simulink model "NarwhaleSimscape"  (R2021b)
settings: Solver=VariableStepAuto  StartTime=0.0  StopTime=12  FixedStep=10^-3  RelTol=1e-3
undefined symbols (not defined in the file): X, Y, Z
libraries: nesl_utility x34, sm_lib x28, slpidlib x5
(part 1 of 3)
settings Model: Creator=matas  LastModifiedBy=matas
settings SolverCC: AlgebraicLoopSolver=TrustRegion
settings DebuggingCC: SFMachineParentedDataDiag=warning

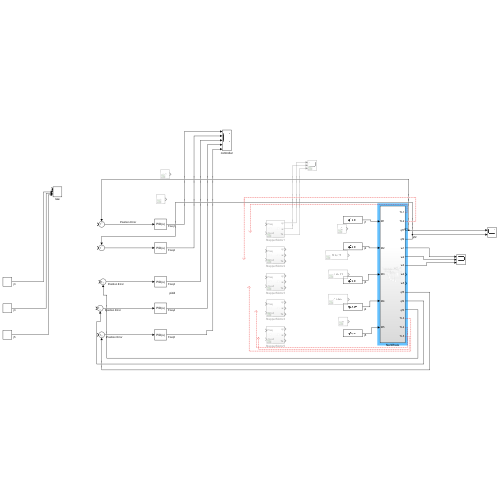
[thumbnail: Simulink's stored preview of the top-level diagram]
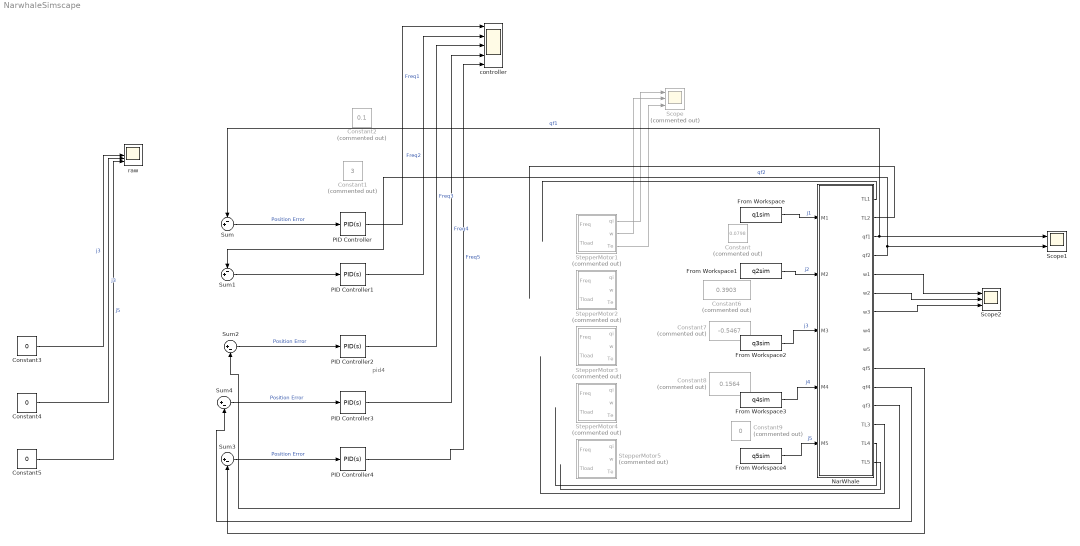
== system NarwhaleSimscape ==
  note: pid4
  Constant : Constant  Commented=on  Value=0.0798
  Constant1 : Constant  Commented=on  Value=3
  Constant2 : Constant  Commented=on  Value=0.1
  Constant3 : Constant  Value=0
  Constant4 : Constant  Value=0
  Constant5 : Constant  Value=0
  Constant6 : Constant  Commented=on  Value=0.3903
  Constant7 : Constant  Commented=on  Value=-0.5467
  Constant8 : Constant  Commented=on  Value=0.1564
  Constant9 : Constant  Commented=on  Value=0
  From Workspace : FromWorkspace  VariableName=q1sim
  From Workspace1 : FromWorkspace  VariableName=q2sim
  From Workspace2 : FromWorkspace  VariableName=q3sim
  From Workspace3 : FromWorkspace  VariableName=q4sim
  From Workspace4 : FromWorkspace  VariableName=q5sim
  NarWhale : Subsystem
  PID Controller : slpidlib/PID Controller  Controller=PID  Form=Parallel  TimeDomain=Continuous-time  UseExternalTs=off  SampleTime=-1  IntegratorMethod=Forward Euler  FilterMethod=Forward Euler  ControllerParametersSource=internal  P=8  I=1  D=0.05  UseFilter=on  N=100  TunerSelectOption=Transfer Function Based (PID Tuner App)  InitialConditionSource=internal  InitialConditionForIntegrator=0  InitialConditionForFilter=0  DifferentiatorICPrevScaledInput=0  ExternalReset=none  TrackingMode=off  Kt=1  LimitOutput=off  SatLimitsSource=internal  UpperSaturationLimit=inf  LowerSaturationLimit=-inf  LinearizeAsGain=on  AntiWindupMode=none  Kb=1  POutMin=[]  POutMax=[]  IOutMin=[]  IOutMax=[]  DOutMin=[]  DOutMax=[]  NOutMin=[]  NOutMax=[]  SumOutMin=[]  SumOutMax=[]  SaturationOutMin=[]  SaturationOutMax=[]  PParamMin=[]  PParamMax=[]  IParamMin=[]  IParamMax=[]  DParamMin=[]  DParamMax=[]  NParamMin=[]  NParamMax=[]  KbParamMin=[]  KbParamMax=[]  KtParamMin=[]  KtParamMax=[]  KbOutMin=[]  KbOutMax=[]  KtOutMin=[]  KtOutMax=[]  IntegratorOutMin=[]  IntegratorOutMax=[]  FilterOutMin=[]  FilterOutMax=[]  SumI1OutMin=[]  SumI1OutMax=[]  SumI2OutMin=[]  SumI2OutMax=[]  SumI3OutMin=[]  SumI3OutMax=[]  SumI4OutMin=[]  SumI4OutMax=[]  SumDOutMin=[]  SumDOutMax=[]  DifferentiatorOutMin=[]  DifferentiatorOutMax=[]  FilterDiffOutCoefMin=[]  FilterDiffOutCoefMax=[]  ReciprocalOutMin=[]  ReciprocalOutMax=[]  SumDenOutMin=[]  SumDenOutMax=[]  SumNumOutMin=[]  SumNumOutMax=[]  DivideOutMin=[]  DivideOutMax=[]  UdiffTsProdOutMin=[]  UdiffTsProdOutMax=[]  NTsProdOutMin=[]  NTsProdOutMax=[]  UintegralTsProdOutMin=[]  UintegralTsProdOutMax=[]  UngainTsProdOutMin=[]  UngainTsProdOutMax=[]  IntegratorContinuousStateAttributes=''  IntegratorStateMustResolveToSignalObject=off  IntegratorRTWStateStorageClass=Auto  FilterContinuousStateAttributes=''  FilterStateMustResolveToSignalObject=off  FilterRTWStateStorageClass=Auto  ParallelPVariant=InternalParameters  IdealPVariant=Disabled  IVariant=InternalParameters  DVariant=InternalParameters  IntegratorVariant=Continuous  SatVariant=Disabled  AWVariant=Passthrough  PCopyVariant=Disabled  TRVariant=Disabled  FdbkBlocksVariant=Forward  IdealPFdbkVariant=Disabled  SatFdbkVariant=Disabled  DerivativeFilterVariant=ContFilter  NVariant=InternalParameters  NCopyVariant=Disabled  FilterICVariant=InternalICsFilter  IntegratorICVariant=InternalICs  ExternalResetVariant=Disabled  TRSumVariant=Passthrough  SumFdbkVariant=Disabled  SumVariant=Sum_PID  TsampFilterVariant=InternalTs  TsampNgainVariant=Passthrough  TsampIntegralVariant=Passthrough  ExternalSaturationOutDataTypeStr=Inherit: Same as second input
  PID Controller{1..4} (4 alike) : slpidlib/PID Controller  Controller=PID  Form=Parallel  TimeDomain=Continuous-time  UseExternalTs=off  SampleTime=-1  IntegratorMethod=Forward Euler  FilterMethod=Forward Euler  ControllerParametersSource=internal  P=8  I=1  D=0.5  UseFilter=on  N=100  TunerSelectOption=Transfer Function Based (PID Tuner App)  InitialConditionSource=internal  InitialConditionForIntegrator=0  InitialConditionForFilter=0  DifferentiatorICPrevScaledInput=0  ExternalReset=none  TrackingMode=off  Kt=1  LimitOutput=off  SatLimitsSource=internal  UpperSaturationLimit=inf  LowerSaturationLimit=-inf  LinearizeAsGain=on  AntiWindupMode=none  Kb=1  POutMin=[]  POutMax=[]  IOutMin=[]  IOutMax=[]  DOutMin=[]  DOutMax=[]  NOutMin=[]  NOutMax=[]  SumOutMin=[]  SumOutMax=[]  SaturationOutMin=[]  SaturationOutMax=[]  PParamMin=[]  PParamMax=[]  IParamMin=[]  IParamMax=[]  DParamMin=[]  DParamMax=[]  NParamMin=[]  NParamMax=[]  KbParamMin=[]  KbParamMax=[]  KtParamMin=[]  KtParamMax=[]  KbOutMin=[]  KbOutMax=[]  KtOutMin=[]  KtOutMax=[]  IntegratorOutMin=[]  IntegratorOutMax=[]  FilterOutMin=[]  FilterOutMax=[]  SumI1OutMin=[]  SumI1OutMax=[]  SumI2OutMin=[]  SumI2OutMax=[]  SumI3OutMin=[]  SumI3OutMax=[]  SumI4OutMin=[]  SumI4OutMax=[]  SumDOutMin=[]  SumDOutMax=[]  DifferentiatorOutMin=[]  DifferentiatorOutMax=[]  FilterDiffOutCoefMin=[]  FilterDiffOutCoefMax=[]  ReciprocalOutMin=[]  ReciprocalOutMax=[]  SumDenOutMin=[]  SumDenOutMax=[]  SumNumOutMin=[]  SumNumOutMax=[]  DivideOutMin=[]  DivideOutMax=[]  UdiffTsProdOutMin=[]  UdiffTsProdOutMax=[]  NTsProdOutMin=[]  NTsProdOutMax=[]  UintegralTsProdOutMin=[]  UintegralTsProdOutMax=[]  UngainTsProdOutMin=[]  UngainTsProdOutMax=[]  IntegratorContinuousStateAttributes=''  IntegratorStateMustResolveToSignalObject=off  IntegratorRTWStateStorageClass=Auto  FilterContinuousStateAttributes=''  FilterStateMustResolveToSignalObject=off  FilterRTWStateStorageClass=Auto  ParallelPVariant=InternalParameters  IdealPVariant=Disabled  IVariant=InternalParameters  DVariant=InternalParameters  IntegratorVariant=Continuous  SatVariant=Disabled  AWVariant=Passthrough  PCopyVariant=Disabled  TRVariant=Disabled  FdbkBlocksVariant=Forward  IdealPFdbkVariant=Disabled  SatFdbkVariant=Disabled  DerivativeFilterVariant=ContFilter  NVariant=InternalParameters  NCopyVariant=Disabled  FilterICVariant=InternalICsFilter  IntegratorICVariant=InternalICs  ExternalResetVariant=Disabled  TRSumVariant=Passthrough  SumFdbkVariant=Disabled  SumVariant=Sum_PID  TsampFilterVariant=InternalTs  TsampNgainVariant=Passthrough  TsampIntegralVariant=Passthrough  ExternalSaturationOutDataTypeStr=Inherit: Same as second input
  Scope : Scope  Commented=on  NumInputPorts=3
  Scope1 : Scope  NumInputPorts=2
  Scope2 : Scope  NumInputPorts=3
  StepperMotor1 : Subsystem  Commented=on
  StepperMotor2 : Subsystem  Commented=on
  StepperMotor3 : Subsystem  Commented=on
  StepperMotor4 : Subsystem  Commented=on
  StepperMotor5 : Subsystem  Commented=on
  Sum : Sum  Inputs=-+|
  Sum1 : Sum  Inputs=-+|
  Sum2 : Sum  Inputs=|+-
  Sum3 : Sum  Inputs=|+-
  Sum4 : Sum  Inputs=|+-
  controller : Scope  NumInputPorts=5
  raw : Scope  NumInputPorts=5
  wires:
  StepperMotor1/1(qi) -> Scope/1
  StepperMotor1/2(w) -> Scope/2
  StepperMotor1/3(Te) -> Scope/3
  NarWhale/1(TL1) -> ?
  NarWhale/3(qf1) -> Sum/1, Scope1/1  "qf1"
  Sum/1 -> PID Controller/1  "Position Error"
  PID Controller/1 -> controller/1  "Freq1"
  PID Controller1/1 -> controller/2  "Freq2"
  Sum1/1 -> PID Controller1/1
  NarWhale/4(qf2) -> Scope1/2, Sum1/1  "qf2"
  NarWhale/2(TL2) -> ?
  Sum2/1 -> PID Controller2/1  "Position Error"
  PID Controller2/1 -> controller/3  "Freq3"
  Constant3/1 -> raw/3  "j3"
  Sum4/1 -> PID Controller3/1  "Position Error"
  PID Controller3/1 -> controller/4  "Freq4"
  NarWhale/12(qf3) -> Sum2/2
  NarWhale/11(qf4) -> Sum4/2
  NarWhale/13(TL3) -> ?
  NarWhale/14(TL4) -> ?
  NarWhale/15(TL5) -> ?
  Constant5/1 -> raw/5  "j5"
  Sum3/1 -> PID Controller4/1  "Position Error"
  PID Controller4/1 -> controller/5  "Freq5"
  NarWhale/10(qf5) -> Sum3/2
  Constant4/1 -> raw/4  "j3"
  NarWhale/5(w1) -> Scope2/1
  NarWhale/6(w2) -> Scope2/2
  NarWhale/7(w3) -> Scope2/3
  From Workspace/1 -> NarWhale/1(M1)  "j1"
  From Workspace1/1 -> NarWhale/2(M2)  "j2"
  From Workspace2/1 -> NarWhale/3(M3)  "j3"
  From Workspace3/1 -> NarWhale/4(M4)  "j4"
  From Workspace4/1 -> NarWhale/5(M5)  "j5"

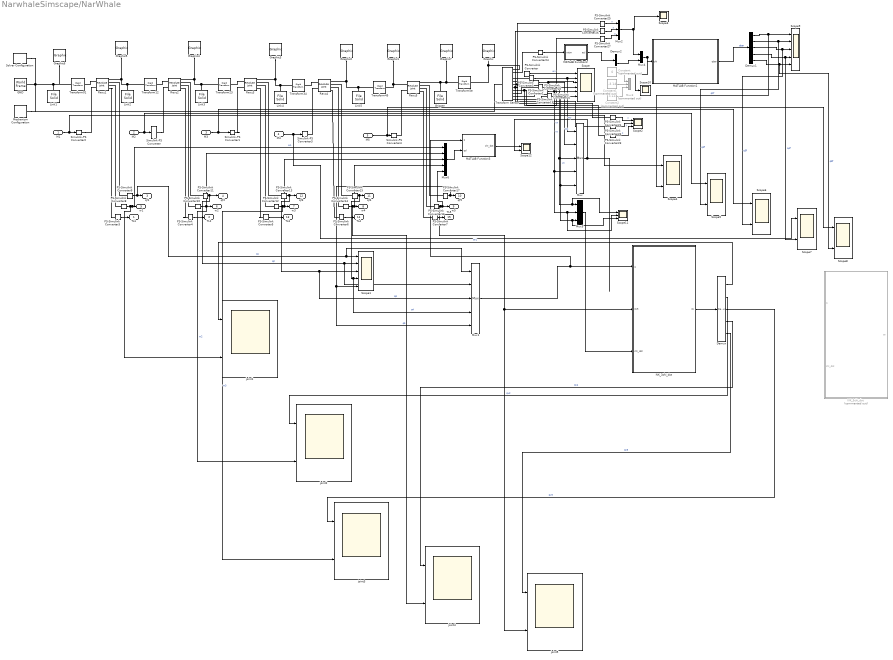
== system NarwhaleSimscape/NarWhale ==
  M1 : Inport
  M2 : Inport  Port=2
  M3 : Inport  Port=3
  M4 : Inport  Port=4
  M5 : Inport  Port=5
  Constant : Constant  Commented=on  Value=0
  Constant1 : Constant  Commented=on  Value=-3.14
  Constant2 : Constant  Commented=on  Value=3.14
  Demux : Demux  Outputs=5
  Demux1 : Demux  Outputs=5
  Demux2 : Demux  Outputs=3
  GND : sm_lib/Frames and Transforms/World Frame
  Graphic : sm_lib/Body Elements/Graphic  GraphicType=Marker  MarkerShape=Frame  MarkerSize=30  GraphicVisPropType=SimpleVisualProperties  GraphicDiffuseColor=[1.0 0.0 0.2]  GraphicSpecularColor=[0.5 0.5 0.5 1.0]  GraphicAmbientColor=[0.15 0.15 0.15 1.0]  GraphicEmissiveColor=[0.0 0.0 0.0 1.0]  GraphicShininess=75  GraphicOpacity=1.0
  Graphic1 : sm_lib/Body Elements/Graphic  GraphicType=Marker  MarkerShape=Frame  MarkerSize=30  GraphicVisPropType=SimpleVisualProperties  GraphicDiffuseColor=[1.0 1.0 0.2]  GraphicSpecularColor=[0.5 0.5 0.5 1.0]  GraphicAmbientColor=[0.15 0.15 0.15 1.0]  GraphicEmissiveColor=[0.0 0.0 0.0 1.0]  GraphicShininess=75  GraphicOpacity=1.0
  Graphic2 : sm_lib/Body Elements/Graphic  GraphicType=Marker  MarkerShape=Frame  MarkerSize=30  GraphicVisPropType=SimpleVisualProperties  GraphicDiffuseColor=[0.2 1.0 0.2]  GraphicSpecularColor=[0.5 0.5 0.5 1.0]  GraphicAmbientColor=[0.15 0.15 0.15 1.0]  GraphicEmissiveColor=[0.0 0.0 0.0 1.0]  GraphicShininess=75  GraphicOpacity=1.0
  Graphic3 : sm_lib/Body Elements/Graphic  GraphicType=Marker  MarkerShape=Frame  MarkerSize=30  GraphicVisPropType=SimpleVisualProperties  GraphicDiffuseColor=[0.2 0.2 1.0]  GraphicSpecularColor=[0.5 0.5 0.5 1.0]  GraphicAmbientColor=[0.15 0.15 0.15 1.0]  GraphicEmissiveColor=[0.0 0.0 0.0 1.0]  GraphicShininess=75  GraphicOpacity=1.0
  Graphic4 : sm_lib/Body Elements/Graphic  GraphicType=Marker  MarkerShape=Frame  MarkerSize=30  GraphicVisPropType=SimpleVisualProperties  GraphicDiffuseColor=[0.6 0.0 1.0]  GraphicSpecularColor=[0.5 0.5 0.5 1.0]  GraphicAmbientColor=[0.15 0.15 0.15 1.0]  GraphicEmissiveColor=[0.0 0.0 0.0 1.0]  GraphicShininess=75  GraphicOpacity=1.0
  Graphic5 : sm_lib/Body Elements/Graphic  GraphicType=Marker  MarkerShape=Frame  MarkerSize=30  GraphicVisPropType=SimpleVisualProperties  GraphicDiffuseColor=[1.0 1.0 1.0]  GraphicSpecularColor=[0.5 0.5 0.5 1.0]  GraphicAmbientColor=[0.15 0.15 0.15 1.0]  GraphicEmissiveColor=[0.0 0.0 0.0 1.0]  GraphicShininess=75  GraphicOpacity=1.0
  Graphic6 : sm_lib/Body Elements/Graphic  GraphicType=Marker  MarkerShape=Frame  MarkerSize=30  GraphicVisPropType=SimpleVisualProperties  GraphicDiffuseColor=[1.0 0.0 1.0]  GraphicSpecularColor=[0.5 0.5 0.5 1.0]  GraphicAmbientColor=[0.15 0.15 0.15 1.0]  GraphicEmissiveColor=[0.0 0.0 0.0 1.0]  GraphicShininess=75  GraphicOpacity=1.0
  Graphic7 : sm_lib/Body Elements/Graphic  GraphicType=Marker  MarkerShape=Frame  MarkerSize=30  GraphicVisPropType=SimpleVisualProperties  GraphicDiffuseColor=[0.4941 0.1843 0.5569]  GraphicSpecularColor=[0.5 0.5 0.5 1.0]  GraphicAmbientColor=[0.15 0.15 0.15 1.0]  GraphicEmissiveColor=[0.0 0.0 0.0 1.0]  GraphicShininess=75  GraphicOpacity=1.0
  Gripper : sm_lib/Body Elements/File Solid  ExtGeomFileName=C:\Users\matas\Documents\GitHub\Module89-Frab5-G3\Matlabscript_simscape\Simscape\NarwhaleCAD\GripperASM.STL  UnitType=Custom  ExtGeomFileUnits=mm  StepReaderType=HEX  ExportConvexHullGeometry=off  InertiaType=Custom  Mass=0.69041  MassUnits=kg  CenterOfMass=[3.8 0.1 197.24]  CenterOfMassUnits=mm  MomentsOfInertia=[17952.2303 19894.8925 4557.2173]  MomentsOfInertiaUnits=g*cm^2  ProductsOfInertia="[-45.0059 -1280.1589  8.8427]"  ProductsOfInertiaUnits=g*cm^2  BasedOnType=DensityFromFile  Density=1000  DensityUnits=kg/m^3  DoExposeReferenceFrame=on  SerializedFrames=<Frames/>  GraphicType=FromGeometry  MarkerShape=Sphere  MarkerSize=10  GraphicVisPropType=SimpleVisualProperties  GraphicDiffuseColor=[0.5 0.5 0.5]  GraphicSpecularColor=[0.5 0.5 0.5 1.0]  GraphicAmbientColor=[0.15 0.15 0.15 1.0]  GraphicEmissiveColor=[0.0 0.0 0.0 1.0]  GraphicShininess=75  GraphicOpacity=1.0
  IVK_3chi_dot : MATLAB Function  TreatAsAtomicUnit=on
  IVK_5chi_dot : MATLAB Function  Commented=on  TreatAsAtomicUnit=on
  Link1 : sm_lib/Body Elements/File Solid  ExtGeomFileName=C:\Users\matas\Documents\GitHub\Module89-Frab5-G3\Matlabscript_simscape\Simscape\NarwhaleCAD\asm_J1.STL  UnitType=Custom  ExtGeomFileUnits=mm  StepReaderType=HEX  ExportConvexHullGeometry=off  InertiaType=Custom  Mass=4.4  MassUnits=kg  CenterOfMass=[-62.94 0.00 77.26]  CenterOfMassUnits=mm  MomentsOfInertia=[233653.95 370833.8212 478183.0941]  MomentsOfInertiaUnits=g*cm^2  ProductsOfInertia=[-8.5995 11773.7055 -0.9031]  ProductsOfInertiaUnits=g*cm^2  BasedOnType=DensityFromFile  Density=1000  DensityUnits=kg/m^3  DoExposeReferenceFrame=on  SerializedFrames=<Frames/>  GraphicType=FromGeometry  MarkerShape=Sphere  MarkerSize=10  GraphicVisPropType=SimpleVisualProperties  GraphicDiffuseColor=[0.5 0.5 0.5]  GraphicSpecularColor=[0.5 0.5 0.5 1.0]  GraphicAmbientColor=[0.15 0.15 0.15 1.0]  GraphicEmissiveColor=[0.0 0.0 0.0 1.0]  GraphicShininess=75  GraphicOpacity=1.0
  Link2 : sm_lib/Body Elements/File Solid  ExtGeomFileName=C:\Users\matas\Documents\GitHub\Module89-Frab5-G3\Matlabscript_simscape\Simscape\NarwhaleCAD\link1.STL  UnitType=Custom  ExtGeomFileUnits=mm  StepReaderType=HEX  ExportConvexHullGeometry=off  InertiaType=Custom  Mass=3.0358  MassUnits=kg  CenterOfMass=[-43.29 -2.02 -88.16]  CenterOfMassUnits=mm  MomentsOfInertia=[97169.4169 112815.4665 119641.6148]  MomentsOfInertiaUnits=g*cm^2  ProductsOfInertia=[13604.2243 136476.2489 6464.8471]  ProductsOfInertiaUnits=g*cm^2  BasedOnType=DensityFromFile  Density=1000  DensityUnits=kg/m^3  DoExposeReferenceFrame=on  SerializedFrames=<Frames/>  GraphicType=FromGeometry  MarkerShape=Sphere  MarkerSize=10  GraphicVisPropType=FromFileVisualProperties  GraphicDiffuseColor=[0.5 0.5 0.5]  GraphicSpecularColor=[0.5 0.5 0.5 1.0]  GraphicAmbientColor=[0.15 0.15 0.15 1.0]  GraphicEmissiveColor=[0.0 0.0 0.0 1.0]  GraphicShininess=75  GraphicOpacity=1.0
  Link3 : sm_lib/Body Elements/File Solid  ExtGeomFileName=C:\Users\matas\Documents\GitHub\Module89-Frab5-G3\Matlabscript_simscape\Simscape\NarwhaleCAD\link2.STL  UnitType=Custom  ExtGeomFileUnits=mm  StepReaderType=HEX  ExportConvexHullGeometry=off  InertiaType=Custom  Mass=2.0778  MassUnits=kg  CenterOfMass=[162 -0.02 8.59]  CenterOfMassUnits=mm  MomentsOfInertia=[24739.1072 311541.7518 294173.41]  MomentsOfInertiaUnits=g*cm^2  ProductsOfInertia=[-387.45 21752.3776 353.8205]  ProductsOfInertiaUnits=g*cm^2  BasedOnType=DensityFromFile  Density=1000  DensityUnits=kg/m^3  DoExposeReferenceFrame=on  SerializedFrames=<Frames/>  GraphicType=FromGeometry  MarkerShape=Sphere  MarkerSize=10  GraphicVisPropType=FromFileVisualProperties  GraphicDiffuseColor=[0.5 0.5 0.5]  GraphicSpecularColor=[0.5 0.5 0.5 1.0]  GraphicAmbientColor=[0.15 0.15 0.15 1.0]  GraphicEmissiveColor=[0.0 0.0 0.0 1.0]  GraphicShininess=75  GraphicOpacity=1.0
  Link4 : sm_lib/Body Elements/File Solid  ExtGeomFileName=C:\Users\matas\Documents\GitHub\Module89-Frab5-G3\Matlabscript_simscape\Simscape\NarwhaleCAD\link3.STL  UnitType=Custom  ExtGeomFileUnits=mm  StepReaderType=HEX  ExportConvexHullGeometry=off  InertiaType=Custom  Mass=1.43881  MassUnits=kg  CenterOfMass=[-175.56 0.06 -6.33]  CenterOfMassUnits=mm  MomentsOfInertia=[16069.2959 173755.3840 164253.8860]  MomentsOfInertiaUnits=g*cm^2  ProductsOfInertia="[-41.6776 3243.5212  -172.4909]"  ProductsOfInertiaUnits=g*cm^2  BasedOnType=DensityFromFile  Density=1000  DensityUnits=kg/m^3  DoExposeReferenceFrame=on  SerializedFrames=<Frames/>  GraphicType=FromGeometry  MarkerShape=Sphere  MarkerSize=10  GraphicVisPropType=FromFileVisualProperties  GraphicDiffuseColor=[0.5 0.5 0.5]  GraphicSpecularColor=[0.5 0.5 0.5 1.0]  GraphicAmbientColor=[0.15 0.15 0.15 1.0]  GraphicEmissiveColor=[0.0 0.0 0.0 1.0]  GraphicShininess=75  GraphicOpacity=1.0
  Link5 : sm_lib/Body Elements/File Solid  ExtGeomFileName=C:\Users\matas\Documents\GitHub\Module89-Frab5-G3\Matlabscript_simscape\Simscape\NarwhaleCAD\J5_Asm.STL  UnitType=Custom  ExtGeomFileUnits=mm  StepReaderType=HEX  ExportConvexHullGeometry=off  InertiaType=Custom  Mass=0.354  MassUnits=kg  CenterOfMass=[-1.28 49.13 0.00]  CenterOfMassUnits=mm  MomentsOfInertia=[6817.7645 2848.9265 5884.7291]  MomentsOfInertiaUnits=g*cm^2  ProductsOfInertia="[-0.2087 1.8247  -13.0414]"  ProductsOfInertiaUnits=g*cm^2  BasedOnType=DensityFromFile  Density=1000  DensityUnits=kg/m^3  DoExposeReferenceFrame=on  SerializedFrames=<Frames/>  GraphicType=FromGeometry  MarkerShape=Sphere  MarkerSize=10  GraphicVisPropType=SimpleVisualProperties  GraphicDiffuseColor=[0.5 0.5 0.5]  GraphicSpecularColor=[0.5 0.5 0.5 1.0]  GraphicAmbientColor=[0.15 0.15 0.15 1.0]  GraphicEmissiveColor=[0.0 0.0 0.0 1.0]  GraphicShininess=75  GraphicOpacity=1.0
  MATLAB Function1 : MATLAB Function  TreatAsAtomicUnit=on
  MATLAB Function2 : MATLAB Function  TreatAsAtomicUnit=on
  MATLAB Function3 : MATLAB Function  TreatAsAtomicUnit=on
  Mechanism Configuration : sm_lib/Utilities/Mechanism Configuration  UniformGravity=Constant  GravityVector=[0 0 -9.80665]  GravityUnits=m/s^2  LinearizationDelta=0.001  JointModeTransitionNonlinearIterations=2
  Mux : Mux  Inputs=5
  Mux1 : Mux  Inputs=5
  Mux2 : Mux  Inputs=3
  Mux3 : Mux  Commented=on  Inputs=3
  Mux4 : Mux  Inputs=2
  Mux5 : Mux  Inputs=3
  Mux6 : Mux  Inputs=5
  PS-Simulink Converter{,1..27} (28 alike) : nesl_utility/PS-Simulink Converter  PhysicalDomain=network_engine_domain  SubClassName=ps_output  LeftPortType=input  RightPortType=output  PseudoPeriodic=off  Frequencies=[]  Unit=inherit  AffineConversion=off
      settings: SourceProductBaseCode=PW,SS
  Revz{1..5} (5 alike) : sm_lib/Joints/Revolute Joint  JointMode=Normal  SenseConstraintForce=off  SenseConstraintForceX=off  SenseConstraintForceY=off  SenseConstraintForceZ=off  SenseConstraintTorque=off  SenseConstraintTorqueX=off  SenseConstraintTorqueY=off  SenseConstraintTorqueZ=off  SenseTotalForce=off  SenseTotalForceX=off  SenseTotalForceY=off  SenseTotalForceZ=off  SenseTotalTorque=off  SenseTotalTorqueX=off  SenseTotalTorqueY=off  SenseTotalTorqueZ=off  CompositeWrenchDir=FollowerOnBase  CompositeWrenchFrame=BaseFrame  EquilibriumPosition=0  EquilibriumPositionUnits=deg  SpringStiffness=0  SpringStiffnessUnits=N*m/deg  DampingCoefficient=0  DampingCoefficientUnits=N*m/(deg/s)  TorqueActuationMode=ComputedTorque  MotionActuationMode=InputMotion  SensePosition=on  SenseVelocity=on  SenseAcceleration=off  SenseTorqueForce=on  SenseLowerLimitTorqueForce=off  SenseUpperLimitTorqueForce=off  LowerLimitSpecify=off  LowerLimitBound=-90  LowerLimitBoundUnits=deg  LowerLimitStiffness=1e4  LowerLimitStiffnessUnits=N*m/deg  LowerLimitDamping=10  LowerLimitDampingUnits=N*m/(deg/s)  LowerLimitTransitionRegionWidth=0.1  LowerLimitTransitionRegionWidthUnits=deg  UpperLimitSpecify=off  UpperLimitBound=90  UpperLimitBoundUnits=deg  UpperLimitStiffness=1e4  UpperLimitStiffnessUnits=N*m/deg  UpperLimitDamping=10  UpperLimitDampingUnits=N*m/(deg/s)  UpperLimitTransitionRegionWidth=0.1  UpperLimitTransitionRegionWidthUnits=deg  PositionTargetSpecify=off  PositionTargetPriority=High  PositionTargetValue=0  PositionTargetValueUnits=deg  VelocityTargetSpecify=off  VelocityTargetPriority=High  VelocityTargetValue=0  VelocityTargetValueUnits=deg/s
  Scope : Scope  NumInputPorts=6
  Scope1 : Scope  NumInputPorts=5
  Scope10 : Scope
  Scope11 : Scope  NumInputPorts=3
  Scope{4..8,12} (6 alike) : Scope  NumInputPorts=2
  Scope2 : Scope  NumInputPorts=3
  Scope3 : Scope
  Scope9 : Scope  NumInputPorts=5
  Simulink-PS Converter : nesl_utility/Simulink-PS Converter  PhysicalDomain=network_engine_domain  SubClassName=ps_input  LeftPortType=input  RightPortType=output  PseudoPeriodic=off  Frequencies=[]  NoiseDistribution=none  NoiseParameters=[]  Unit=1  AffineConversion=off  FilteringAndDerivatives=filter  SimscapeFilterOrder=2  InputFilterTimeConstant=0.001  UdotUserProvided=1
      settings: SourceProductBaseCode=PW,SS
  Simulink-PS Converter{1..4} (4 alike) : nesl_utility/Simulink-PS Converter  PhysicalDomain=network_engine_domain  SubClassName=ps_input  LeftPortType=input  RightPortType=output  PseudoPeriodic=off  Frequencies=[]  NoiseDistribution=none  NoiseParameters=[]  Unit=1  AffineConversion=off  FilteringAndDerivatives=filter  SimscapeFilterOrder=2  InputFilterTimeConstant=0.001  UdotUserProvided=0
      settings: SourceProductBaseCode=PW,SS
  Solver Configuration : nesl_utility/Solver Configuration  PhysicalDomain=network_engine_domain  SubClassName=solver  LeftPortType=input  RightPortType=generic  Tones=[]  Harmonics=[]  SimulateNoise=off  Profile=off  UseLocalSampling=off  EnableSwitchedLinearOptims=on  FrequencyDomain=off  UseCCode=off  RelTol=0.001  AbsTol=1e-06  MinStep=1e-09  ToWorkspace=off  RevertToSquareIcSolve=off  NumHomotopyIterations=100  PhasorMode=off  PhasorModeNumHarmonics=1  DoDC=off  ResidualTolerance=1e-09  UseLocalSolver=off  LocalSolverChoice=NE_BACKWARD_EULER_ADVANCER  LocalSolverSampleTime=0.001  DoFixedCost=off  MaxNonlinIter=3  MaxModeIter=2  ComputeImpulses=off  ImpulseIterations=2  LinearAlgebra=auto  EquationFormulation=NE_TIME_EF  DelaysMemoryBudget=1024  AutomaticFiltering=on  FilteringTimeConstant=0.001  PartitionStorageMethod=AS_NEEDED  PartitionMemoryBudget=1024  PartitionMethod=ROBUST
      settings: SourceProductBaseCode=PW,SS
  Transform Sensor : sm_lib/Frames and Transforms/Transform Sensor  MeasurementFrame=World  SenseAngle=off  SenseAxis=off  SenseAngle1=off  SenseAngle2=off  SenseAngle3=off  SenseQ=off  SenseR=on  SenseOmegaX=on  SenseOmegaY=on  SenseOmegaZ=on  SenseOmega1=off  SenseOmega2=off  SenseOmega3=off  SenseQDot=off  SenseRDot=off  SenseAlphaX=off  SenseAlphaY=off  SenseAlphaZ=off  SenseAlpha1=off  SenseAlpha2=off  SenseAlpha3=off  SenseQDDot=off  SenseRDDot=off  SenseX=on  SenseY=on  SenseZ=on  SenseRad=off  SenseAzim=off  SenseDist=off  SenseInc=off  SenseXDot=on  SenseYDot=on  SenseZDot=on  SenseRadDot=off  SenseAzimDot=off  SenseDistDot=off  SenseIncDot=off  SenseXDDot=off  SenseYDDot=off  SenseZDDot=off  SenseRadDDot=off  SenseAzimDDot=off  SenseDistDDot=off  SenseIncDDot=off
  Transform01 : sm_lib/Frames and Transforms/Rigid Transform  TranslationMethod=StandardAxis  TranslationStandardOffset=0.29589  TranslationLengthUnit=m  TranslationStandardAxis=+Z  TranslationCartesianOffset=[0 0 0]  TranslationROffset=0  TranslationROffsetUnits=m  TranslationZOffset=0  TranslationZOffsetUnits=m  TranslationThetaOffset=0  TranslationThetaOffsetUnits=deg  RotationMethod=None  RotationAngleUnits=deg  RotationStandardAxis=+Z  RotationAngle=0.0  RotationArbitraryAxis=[0 0 1]  FollAlignAxisA=+X  BaseAlignAxisA=+Y  FollAlignAxisB=+Y  BaseAlignAxisB=+Z  RotationSequenceAxes=FollowerAxes  RotationSequence=XYX  RotationSequenceAngles=[0 0 0]  RotationSequenceAnglesUnits=deg  RotationMatrix=[1 0 0; 0 1 0; 0 0 1]
  Transform12 : sm_lib/Frames and Transforms/Rigid Transform  TranslationMethod=StandardAxis  TranslationStandardOffset=0.0200  TranslationLengthUnit=m  TranslationStandardAxis=+X  TranslationCartesianOffset=[0 0 0]  TranslationROffset=0  TranslationROffsetUnits=m  TranslationZOffset=0  TranslationZOffsetUnits=m  TranslationThetaOffset=0  TranslationThetaOffsetUnits=deg  RotationMethod=AlignedAxes  RotationAngleUnits=deg  RotationStandardAxis=+Z  RotationAngle=0.0  RotationArbitraryAxis=[0 0 1]  FollAlignAxisA=+X  BaseAlignAxisA=+Z  FollAlignAxisB=-Y  BaseAlignAxisB=+X  RotationSequenceAxes=BaseAxes  RotationSequence=XYX  RotationSequenceAngles=[0 0 0]  RotationSequenceAnglesUnits=deg  RotationMatrix=[1 0 0; 0 1 0; 0 0 1]
  Transform23 : sm_lib/Frames and Transforms/Rigid Transform  TranslationMethod=StandardAxis  TranslationStandardOffset=0.380  TranslationLengthUnit=m  TranslationStandardAxis=+X  TranslationCartesianOffset=[0 0 0]  TranslationROffset=0  TranslationROffsetUnits=m  TranslationZOffset=0  TranslationZOffsetUnits=m  TranslationThetaOffset=0  TranslationThetaOffsetUnits=deg  RotationMethod=AlignedAxes  RotationAngleUnits=deg  RotationStandardAxis=+Z  RotationAngle=0.0  RotationArbitraryAxis=[0 0 1]  FollAlignAxisA=+Z  BaseAlignAxisA=+Z  FollAlignAxisB=+Y  BaseAlignAxisB=+X  RotationSequenceAxes=FollowerAxes  RotationSequence=XYX  RotationSequenceAngles=[0 0 0]  RotationSequenceAnglesUnits=deg  RotationMatrix=[1 0 0; 0 1 0; 0 0 1]
  Transform34 : sm_lib/Frames and Transforms/Rigid Transform  TranslationMethod=StandardAxis  TranslationStandardOffset=0.380  TranslationLengthUnit=m  TranslationStandardAxis=+X  TranslationCartesianOffset=[0 0 0]  TranslationROffset=0  TranslationROffsetUnits=m  TranslationZOffset=0  TranslationZOffsetUnits=m  TranslationThetaOffset=0  TranslationThetaOffsetUnits=deg  RotationMethod=None  RotationAngleUnits=deg  RotationStandardAxis=+Z  RotationAngle=0.0  RotationArbitraryAxis=[0 0 1]  FollAlignAxisA=+Z  BaseAlignAxisA=+Z  FollAlignAxisB=+Y  BaseAlignAxisB=+X  RotationSequenceAxes=FollowerAxes  RotationSequence=XYX  RotationSequenceAngles=[0 0 0]  RotationSequenceAnglesUnits=deg  RotationMatrix=[1 0 0; 0 1 0; 0 0 1]
  Transform45 : sm_lib/Frames and Transforms/Rigid Transform  TranslationMethod=None  TranslationStandardOffset=380  TranslationLengthUnit=mm  TranslationStandardAxis=+X  TranslationCartesianOffset=[0 0 0]  TranslationROffset=0  TranslationROffsetUnits=m  TranslationZOffset=0  TranslationZOffsetUnits=m  TranslationThetaOffset=0  TranslationThetaOffsetUnits=deg  RotationMethod=StandardAxis  RotationAngleUnits=rad  RotationStandardAxis=+X  RotationAngle=pi/2  RotationArbitraryAxis=[0 0 1]  FollAlignAxisA=+Z  BaseAlignAxisA=+Z  FollAlignAxisB=+Y  BaseAlignAxisB=+X  RotationSequenceAxes=FollowerAxes  RotationSequence=XYX  RotationSequenceAngles=[0 0 0]  RotationSequenceAnglesUnits=deg  RotationMatrix=[1 0 0; 0 1 0; 0 0 1]
  Transform5e : sm_lib/Frames and Transforms/Rigid Transform  TranslationMethod=StandardAxis  TranslationStandardOffset=0.269  TranslationLengthUnit=m  TranslationStandardAxis=+Z  TranslationCartesianOffset=[0 0 0]  TranslationROffset=0  TranslationROffsetUnits=m  TranslationZOffset=0  TranslationZOffsetUnits=m  TranslationThetaOffset=0  TranslationThetaOffsetUnits=deg  RotationMethod=None  RotationAngleUnits=deg  RotationStandardAxis=+X  RotationAngle=90  RotationArbitraryAxis=[0 0 1]  FollAlignAxisA=+Z  BaseAlignAxisA=+Z  FollAlignAxisB=+Y  BaseAlignAxisB=+X  RotationSequenceAxes=FollowerAxes  RotationSequence=XYX  RotationSequenceAngles=[0 0 0]  RotationSequenceAnglesUnits=deg  RotationMatrix=[1 0 0; 0 1 0; 0 0 1]
  joint{1..5} (5 alike) : Scope  NumInputPorts=2
  TL1 : Outport
  TL2 : Outport  Port=2
  qf1 : Outport  Port=3
  qf2 : Outport  Port=4
  w1 : Outport  Port=5
  w2 : Outport  Port=6
  w3 : Outport  Port=7
  w4 : Outport  Port=8
  w5 : Outport  Port=9
  qf5 : Outport  Port=10
  qf4 : Outport  Port=11
  qf3 : Outport  Port=12
  TL3 : Outport  Port=13
  TL4 : Outport  Port=14
  TL5 : Outport  Port=15
  wires:
  PS-Simulink Converter17/1 -> Scope1/5, Mux1/5, qf5/1  "q5"
  PS-Simulink Converter15/1 -> Mux1/4, Scope1/4, qf4/1  "q4"
  PS-Simulink Converter13/1 -> Scope1/3, Mux1/3, qf3/1  "q3"
  PS-Simulink Converter3/1 -> TL1/1
  PS-Simulink Converter14/1 -> Mux6/4, w4/1, joint4/2
  PS-Simulink Converter4/1 -> TL2/1
  PS-Simulink Converter10/1 -> joint2/2, Mux6/2, w2/1  "w2"
  PS-Simulink Converter7/1 -> TL5/1
  PS-Simulink Converter5/1 -> TL3/1
  PS-Simulink Converter12/1 -> joint3/2, Mux6/3, w3/1  "w3"
  PS-Simulink Converter6/1 -> TL4/1
  PS-Simulink Converter11/1 -> Scope1/2, Mux1/2, qf2/1  "q2"
  PS-Simulink Converter9/1 -> Mux1/1, Scope1/1, qf1/1  "q1"
  PS-Simulink Converter16/1 -> Mux6/5, w5/1, IVK_3chi_dot/2(qv5), joint5/2
  PS-Simulink Converter8/1 -> joint1/2, Mux6/1, w1/1  "w1"
  PS-Simulink Converter/1 -> Scope/1  "wx"
  PS-Simulink Converter1/1 -> Mux/1, Scope/2  "wy"
  PS-Simulink Converter2/1 -> Mux/2, Scope/3  "wz"
  PS-Simulink Converter18/1 -> Scope11/1, Mux5/1, Mux/3, Scope/4  "vx"
  PS-Simulink Converter19/1 -> Mux5/2, Scope11/2, Mux/4, Scope/5  "vy"
  PS-Simulink Converter20/1 -> Scope11/3, Mux5/3, Mux/5, Scope/6  "vz"
  M1/1 -> Scope4/1, Simulink-PS Converter2/1
  M2/1 -> Scope5/1, Simulink-PS Converter/1
  M3/1 -> Scope6/1, Simulink-PS Converter1/1
  M4/1 -> Scope7/1, Simulink-PS Converter3/1
  M5/1 -> Scope8/1, Simulink-PS Converter4/1
  Mux/1 -> Scope12/2
  Mux1/1 -> IVK_3chi_dot/1(q), MATLAB Function3/1(q)
  IVK_3chi_dot/1(qv) -> Demux/1
  Demux/1 -> joint1/1  "qv1"
  Demux/2 -> joint2/1  "qv2"
  Demux/3 -> joint3/1  "qv3"
  Demux/4 -> joint4/1  "qv4"
  Demux/5 -> joint5/1  "qv5"
  PS-Simulink Converter21/1 -> Scope2/1  "x"
  PS-Simulink Converter22/1 -> Scope2/2  "y"
  PS-Simulink Converter23/1 -> Scope2/3  "z"
  PS-Simulink Converter24/1 -> MATLAB Function2/1(rotm)
  PS-Simulink Converter25/1 -> Mux2/1  "x"
  PS-Simulink Converter26/1 -> Mux2/2  "y"
  PS-Simulink Converter27/1 -> Mux2/3  "z"
  MATLAB Function1/1(qbar) -> Demux1/1  "qbar"
  Demux1/1 -> Scope4/2, Scope9/1  "q1f"
  Demux1/4 -> Scope7/2, Scope9/4  "q4f"
  Demux1/5 -> Scope8/2, Scope9/5  "q5f"
  Constant/1 -> Mux3/1
  Constant1/1 -> Mux3/2
  Constant2/1 -> Mux3/3
  Mux2/1 -> Mux4/1, Scope3/1
  Demux1/2 -> Scope5/2, Scope9/2  "q2f"
  Demux1/3 -> Scope6/2, Scope9/3  "q3f"
  MATLAB Function2/1(eul) -> Demux2/1
  Demux2/3 -> Mux4/2
  Mux4/1 -> Scope10/1, MATLAB Function1/1(chi)
  Mux5/1 -> IVK_3chi_dot/3(chi_dot)
  Mux6/1 -> MATLAB Function3/2(qd)
  MATLAB Function3/1(chi_dot) -> Scope12/1
  connections:
  PS-Simulink Converter7/LConn1 -- Revz5/RConn4
  PS-Simulink Converter10/LConn1 -- Revz2/RConn3
  PS-Simulink Converter13/LConn1 -- Revz3/RConn2
  Link4/RConn1 -- Revz3/RConn1 -- Graphic3/RConn1 -- Transform34/LConn1
  Simulink-PS Converter/RConn1 -- Revz2/LConn2
  PS-Simulink Converter9/LConn1 -- Revz1/RConn2
  PS-Simulink Converter15/LConn1 -- Revz4/RConn2
  Link2/RConn1 -- Transform12/LConn1 -- Revz1/RConn1 -- Graphic5/RConn1
  Solver Configuration/RConn1 -- Graphic6/RConn1 -- Transform01/LConn1 -- Link1/RConn1 -- Transform Sensor/LConn1 -- Mechanism Configuration/RConn1 -- GND/RConn1
  Graphic/RConn1 -- Transform5e/RConn1 -- Transform Sensor/RConn1
  Revz4/LConn1 -- Transform34/RConn1
  Revz2/LConn1 -- Transform12/RConn1
  PS-Simulink Converter11/LConn1 -- Revz2/RConn2
  Simulink-PS Converter4/RConn1 -- Revz5/LConn2
  PS-Simulink Converter12/LConn1 -- Revz3/RConn3
  Link5/RConn1 -- Transform45/LConn1 -- Revz4/RConn1 -- Graphic2/RConn1
  PS-Simulink Converter5/LConn1 -- Revz3/RConn4
  Simulink-PS Converter1/RConn1 -- Revz3/LConn2
  PS-Simulink Converter8/LConn1 -- Revz1/RConn3
  Revz4/LConn2 -- Simulink-PS Converter3/RConn1
  Revz3/LConn1 -- Transform23/RConn1
  Graphic1/RConn1 -- Revz5/LConn1 -- Transform45/RConn1
  PS-Simulink Converter14/LConn1 -- Revz4/RConn3
  Link3/RConn1 -- Graphic4/RConn1 -- Revz2/RConn1 -- Transform23/LConn1
  PS-Simulink Converter6/LConn1 -- Revz4/RConn4
  Revz1/LConn1 -- Transform01/RConn1
  PS-Simulink Converter17/LConn1 -- Revz5/RConn2
  Simulink-PS Converter2/RConn1 -- Revz1/LConn2
  PS-Simulink Converter4/LConn1 -- Revz2/RConn4
  PS-Simulink Converter16/LConn1 -- Revz5/RConn3
  Revz1/RConn4 -- PS-Simulink Converter3/LConn1
  Transform5e/LConn1 -- Gripper/RConn1 -- Revz5/RConn1 -- Graphic7/RConn1
  PS-Simulink Converter24/LConn1 -- Transform Sensor/RConn2
  Transform Sensor/RConn6 -- PS-Simulink Converter25/LConn1 -- PS-Simulink Converter21/LConn1
  Transform Sensor/RConn7 -- PS-Simulink Converter26/LConn1 -- PS-Simulink Converter22/LConn1
  Transform Sensor/RConn8 -- PS-Simulink Converter23/LConn1 -- PS-Simulink Converter27/LConn1
  Transform Sensor/RConn9 -- PS-Simulink Converter18/LConn1
  Transform Sensor/RConn10 -- PS-Simulink Converter19/LConn1
  Transform Sensor/RConn11 -- PS-Simulink Converter20/LConn1
  Transform Sensor/RConn5 -- PS-Simulink Converter2/LConn1
  Transform Sensor/RConn4 -- PS-Simulink Converter1/LConn1

== system NarwhaleSimscape/StepperMotor1 ==
  Freq : Inport
  Tload : Inport  Port=2
  Pulse Generator : Subsystem
  Stepper Motor Model : Subsystem
  qi : Outport
  w : Outport  Port=2
  Te : Outport  Port=3
  wires:
  Stepper Motor Model/3(Te) -> Te/1  "Te"
  Freq/1 -> Pulse Generator/1(Freq)
  Stepper Motor Model/1(Theta) -> qi/1  "Theta"
  Tload/1 -> Stepper Motor Model/3(Tload)
  Pulse Generator/2(SignalB) -> Stepper Motor Model/2(SignalB)
  Stepper Motor Model/2(W) -> w/1  "W"
  Pulse Generator/1(SignalA) -> Stepper Motor Model/1(SignalA)

== system NarwhaleSimscape/StepperMotor2 ==
  Freq : Inport
  Tload : Inport  Port=2
  Pulse Generator : Subsystem
  Stepper Motor Model : Subsystem
  qi : Outport
  w : Outport  Port=2
  Te : Outport  Port=3
  wires:
  Stepper Motor Model/3(Te) -> Te/1  "Te"
  Freq/1 -> Pulse Generator/1(Freq)
  Stepper Motor Model/1(Theta) -> qi/1  "Theta"
  Tload/1 -> Stepper Motor Model/3(Tload)
  Pulse Generator/2(SignalB) -> Stepper Motor Model/2(SignalB)
  Stepper Motor Model/2(W) -> w/1  "W"
  Pulse Generator/1(SignalA) -> Stepper Motor Model/1(SignalA)

== system NarwhaleSimscape/StepperMotor3 ==
  Freq : Inport
  Tload : Inport  Port=2
  Pulse Generator : Subsystem
  Stepper Motor Model : Subsystem
  qi : Outport
  w : Outport  Port=2
  Te : Outport  Port=3
  wires:
  Stepper Motor Model/3(Te) -> Te/1  "Te"
  Freq/1 -> Pulse Generator/1(Freq)
  Stepper Motor Model/1(Theta) -> qi/1  "Theta"
  Tload/1 -> Stepper Motor Model/3(Tload)
  Pulse Generator/2(SignalB) -> Stepper Motor Model/2(SignalB)
  Stepper Motor Model/2(W) -> w/1  "W"
  Pulse Generator/1(SignalA) -> Stepper Motor Model/1(SignalA)

== system NarwhaleSimscape/StepperMotor4 ==
  Freq : Inport
  Tload : Inport  Port=2
  Pulse Generator : Subsystem
  Stepper Motor Model : Subsystem
  qi : Outport
  w : Outport  Port=2
  Te : Outport  Port=3
  wires:
  Stepper Motor Model/3(Te) -> Te/1  "Te"
  Freq/1 -> Pulse Generator/1(Freq)
  Stepper Motor Model/1(Theta) -> qi/1  "Theta"
  Tload/1 -> Stepper Motor Model/3(Tload)
  Pulse Generator/2(SignalB) -> Stepper Motor Model/2(SignalB)
  Stepper Motor Model/2(W) -> w/1  "W"
  Pulse Generator/1(SignalA) -> Stepper Motor Model/1(SignalA)

== system NarwhaleSimscape/StepperMotor5 ==
  Freq : Inport
  Tload : Inport  Port=2
  Pulse Generator : Subsystem
  Stepper Motor Model : Subsystem
  qi : Outport
  w : Outport  Port=2
  Te : Outport  Port=3
  wires:
  Stepper Motor Model/3(Te) -> Te/1  "Te"
  Freq/1 -> Pulse Generator/1(Freq)
  Stepper Motor Model/1(Theta) -> qi/1  "Theta"
  Tload/1 -> Stepper Motor Model/3(Tload)
  Pulse Generator/2(SignalB) -> Stepper Motor Model/2(SignalB)
  Stepper Motor Model/2(W) -> w/1  "W"
  Pulse Generator/1(SignalA) -> Stepper Motor Model/1(SignalA)

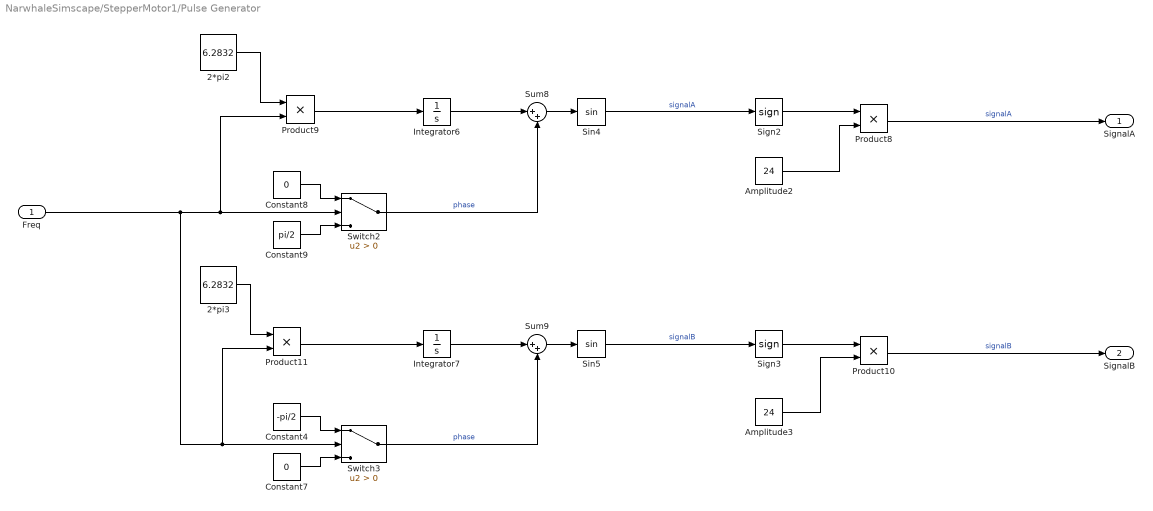
== system NarwhaleSimscape/StepperMotor1/Pulse Generator ==
  Freq : Inport
  2*pi2 : Constant  Value=6.2832
  2*pi3 : Constant  Value=6.2832
  Amplitude2 : Constant  Value=24
  Amplitude3 : Constant  Value=24
  Constant4 : Constant  Value=-pi/2
  Constant7 : Constant  Value=0
  Constant8 : Constant  Value=0
  Constant9 : Constant  Value=pi/2
  Integrator6 : Integrator
  Integrator7 : Integrator
  Product{8..11} (4 alike) : Product
  Sign2 : Signum
  Sign3 : Signum
  Sin4 : Trigonometry
  Sin5 : Trigonometry
  Sum8 : Sum  Inputs=|++
  Sum9 : Sum  Inputs=|++
  Switch2 : Switch  Criteria=u2 > Threshold
  Switch3 : Switch  Criteria=u2 > Threshold
  SignalA : Outport
  SignalB : Outport  Port=2
  wires:
  Product11/1 -> Integrator7/1
  Switch3/1 -> Sum9/2  "phase"
  Sum8/1 -> Sin4/1
  Sign3/1 -> Product10/1
  Integrator7/1 -> Sum9/1
  Freq/1 -> Product11/2, Switch3/2, Product9/2, Switch2/2
  Sin5/1 -> Sign3/1  "signalB"
  Sign2/1 -> Product8/1
  Product10/1 -> SignalB/1  "signalB"
  Product8/1 -> SignalA/1  "signalA"
  Amplitude3/1 -> Product10/2
  Sum9/1 -> Sin5/1
  Amplitude2/1 -> Product8/2
  Integrator6/1 -> Sum8/1
  Constant4/1 -> Switch3/1
  Constant7/1 -> Switch3/3
  2*pi3/1 -> Product11/1
  Switch2/1 -> Sum8/2  "phase"
  Constant9/1 -> Switch2/3
  Constant8/1 -> Switch2/1
  2*pi2/1 -> Product9/1
  Sin4/1 -> Sign2/1  "signalA"
  Product9/1 -> Integrator6/1

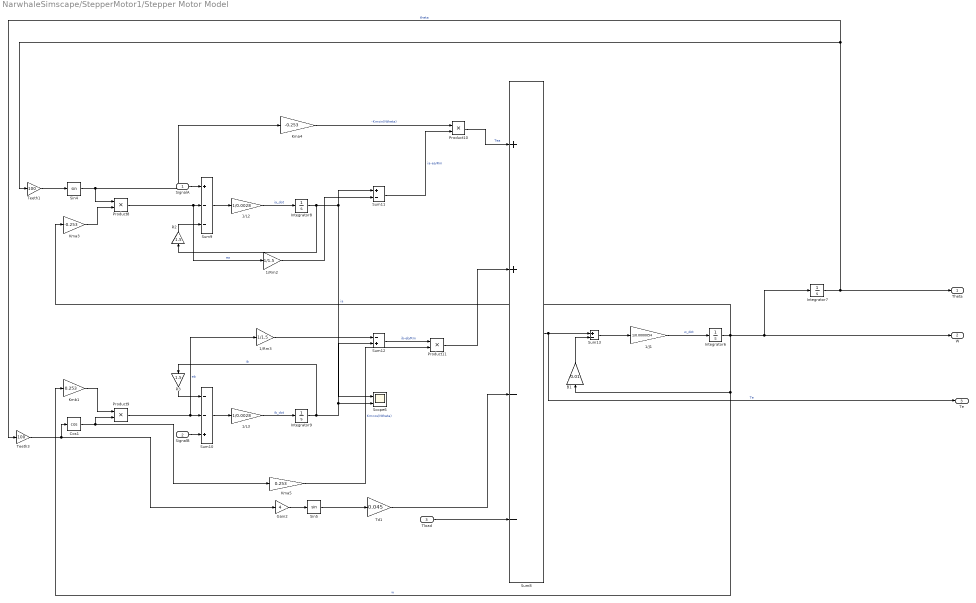
== system NarwhaleSimscape/StepperMotor1/Stepper Motor Model ==
  SignalA : Inport
  SignalB : Inport  Port=2
  Tload : Inport  Port=3
  1/J1 : Gain  Gain=1/0.0000054
  1/L2 : Gain  Gain=1/0.0028
  1/L3 : Gain  Gain=1/0.0028
  1/Rm2 : Gain  Gain=1/1.5
  1/Rm3 : Gain  Gain=1/1.5
  B1 : Gain  Gain=0.01
  Cos1 : Trigonometry  Operator=cos
  Gain2 : Gain  Gain=4
  Integrator{6..9} (4 alike) : Integrator
  Kma3 : Gain  Gain=-0.253
  Kma4 : Gain  Gain=-0.253
  Kma5 : Gain  Gain=0.253
  Kmb1 : Gain  Gain=0.253
  Product{8..11} (4 alike) : Product
  R2 : Gain  Gain=1.5
  R3 : Gain  Gain=1.5
  Scope6 : Scope  NumInputPorts=2
  Sin4 : Trigonometry
  Sin5 : Trigonometry
  Sum10 : Sum  Inputs=--+
  Sum11 : Sum  Inputs=+-
  Sum12 : Sum  Inputs=-+
  Sum13 : Sum  Inputs=+-
  Sum8 : Sum  Inputs=++--
  Sum9 : Sum  Inputs=+--
  Td1 : Gain  Gain=0.045
  Teeth1 : Gain  Gain=100
  Teeth3 : Gain  Gain=100
  Theta : Outport
  W : Outport  Port=2
  Te : Outport  Port=3
  wires:
  Sum10/1 -> 1/L3/1
  1/L3/1 -> Integrator9/1  "ib_dot"
  Cos1/1 -> Kma5/1, Product9/2
  Tload/1 -> Sum8/4
  Gain2/1 -> Sin5/1
  Sum9/1 -> 1/L2/1
  SignalB/1 -> Sum10/3
  Sum13/1 -> 1/J1/1
  Product8/1 -> 1/Rm2/1, Sum9/2  "ea"
  Product11/1 -> Sum8/2
  Teeth3/1 -> Gain2/1, Cos1/1
  SignalA/1 -> Sum9/1
  Sum11/1 -> Product10/2  "ia-ea/Rm"
  1/Rm3/1 -> Sum12/1
  B1/1 -> Sum13/2
  Integrator7/1 -> Theta/1, Teeth1/1, Teeth3/1  "theta"
  Integrator6/1 -> Kmb1/1, B1/1, Kma3/1, W/1, Integrator7/1  "w"
  Sin4/1 -> Kma4/1, Product8/1
  Integrator8/1 -> Scope6/1, Sum11/1, R2/1  "ia"
  R2/1 -> Sum9/3
  Product9/1 -> 1/Rm3/1, Sum10/2  "eb"
  Kma3/1 -> Product8/2
  Sum12/1 -> Product11/1  "ib-eb/Rm"
  1/Rm2/1 -> Sum11/2
  Kmb1/1 -> Product9/1
  Product10/1 -> Sum8/1  "Tea"
  Integrator9/1 -> Scope6/2, Sum12/2, R3/1  "ib"
  Sum8/1 -> Te/1, Sum13/1  "Te"
  1/J1/1 -> Integrator6/1  "w_dot"
  Kma4/1 -> Product10/1  "-Kmsin(Ntheta)"
  Sin5/1 -> Td1/1
  Kma5/1 -> Product11/2  "Kmcos(Ntheta)"
  1/L2/1 -> Integrator8/1  "ia_dot"
  Teeth1/1 -> Sin4/1
  R3/1 -> Sum10/1
  Td1/1 -> Sum8/3

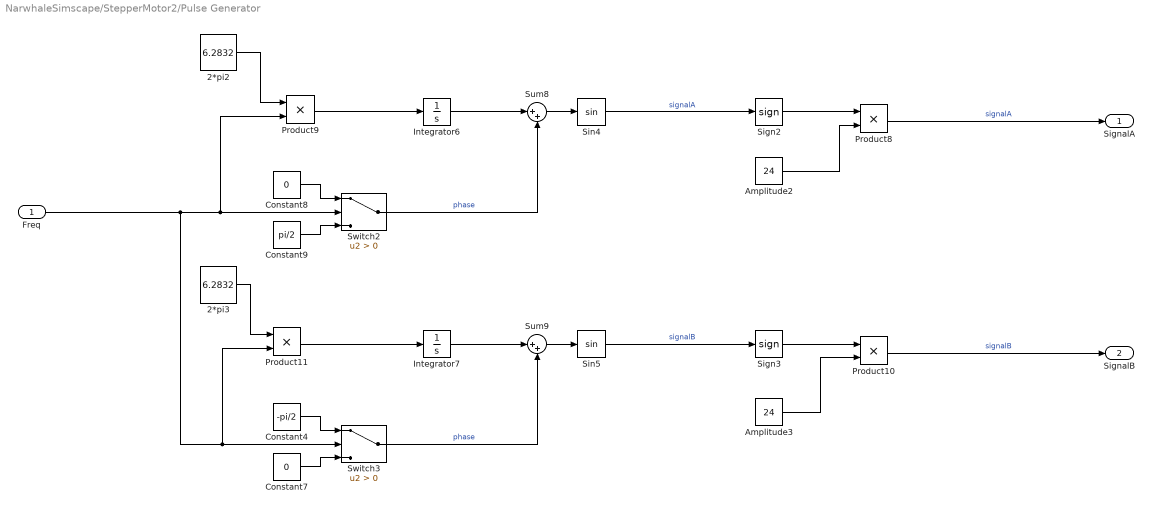
== system NarwhaleSimscape/StepperMotor2/Pulse Generator ==
  Freq : Inport
  2*pi2 : Constant  Value=6.2832
  2*pi3 : Constant  Value=6.2832
  Amplitude2 : Constant  Value=24
  Amplitude3 : Constant  Value=24
  Constant4 : Constant  Value=-pi/2
  Constant7 : Constant  Value=0
  Constant8 : Constant  Value=0
  Constant9 : Constant  Value=pi/2
  Integrator6 : Integrator
  Integrator7 : Integrator
  Product{8..11} (4 alike) : Product
  Sign2 : Signum
  Sign3 : Signum
  Sin4 : Trigonometry
  Sin5 : Trigonometry
  Sum8 : Sum  Inputs=|++
  Sum9 : Sum  Inputs=|++
  Switch2 : Switch  Criteria=u2 > Threshold
  Switch3 : Switch  Criteria=u2 > Threshold
  SignalA : Outport
  SignalB : Outport  Port=2
  wires:
  Product11/1 -> Integrator7/1
  Switch3/1 -> Sum9/2  "phase"
  Sum8/1 -> Sin4/1
  Sign3/1 -> Product10/1
  Integrator7/1 -> Sum9/1
  Freq/1 -> Product11/2, Switch3/2, Product9/2, Switch2/2
  Sin5/1 -> Sign3/1  "signalB"
  Sign2/1 -> Product8/1
  Product10/1 -> SignalB/1  "signalB"
  Product8/1 -> SignalA/1  "signalA"
  Amplitude3/1 -> Product10/2
  Sum9/1 -> Sin5/1
  Amplitude2/1 -> Product8/2
  Integrator6/1 -> Sum8/1
  Constant4/1 -> Switch3/1
  Constant7/1 -> Switch3/3
  2*pi3/1 -> Product11/1
  Switch2/1 -> Sum8/2  "phase"
  Constant9/1 -> Switch2/3
  Constant8/1 -> Switch2/1
  2*pi2/1 -> Product9/1
  Sin4/1 -> Sign2/1  "signalA"
  Product9/1 -> Integrator6/1

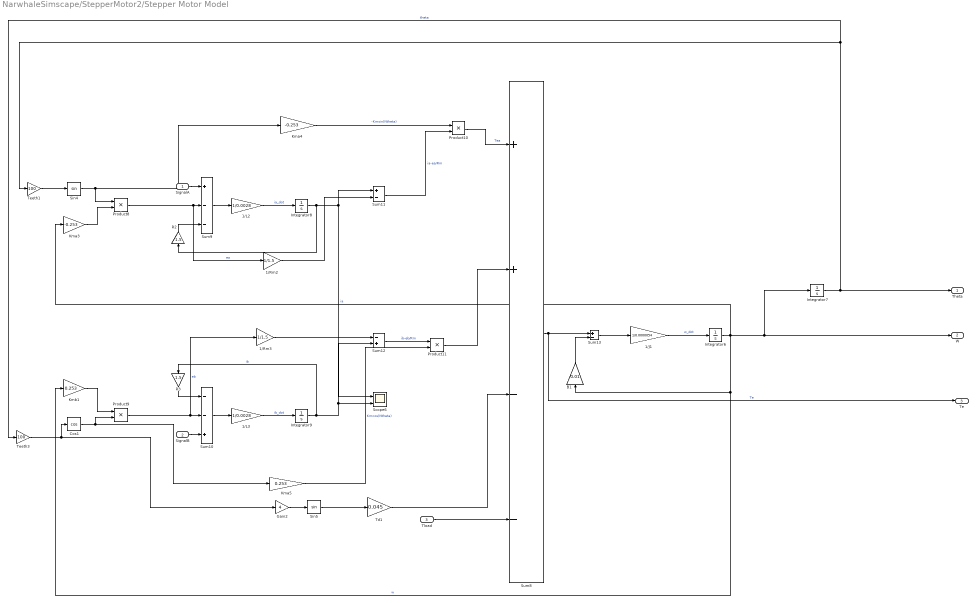
== system NarwhaleSimscape/StepperMotor2/Stepper Motor Model ==
  SignalA : Inport
  SignalB : Inport  Port=2
  Tload : Inport  Port=3
  1/J1 : Gain  Gain=1/0.0000054
  1/L2 : Gain  Gain=1/0.0028
  1/L3 : Gain  Gain=1/0.0028
  1/Rm2 : Gain  Gain=1/1.5
  1/Rm3 : Gain  Gain=1/1.5
  B1 : Gain  Gain=0.01
  Cos1 : Trigonometry  Operator=cos
  Gain2 : Gain  Gain=4
  Integrator{6..9} (4 alike) : Integrator
  Kma3 : Gain  Gain=-0.253
  Kma4 : Gain  Gain=-0.253
  Kma5 : Gain  Gain=0.253
  Kmb1 : Gain  Gain=0.253
  Product{8..11} (4 alike) : Product
  R2 : Gain  Gain=1.5
  R3 : Gain  Gain=1.5
  Scope6 : Scope  NumInputPorts=2
  Sin4 : Trigonometry
  Sin5 : Trigonometry
  Sum10 : Sum  Inputs=--+
  Sum11 : Sum  Inputs=+-
  Sum12 : Sum  Inputs=-+
  Sum13 : Sum  Inputs=+-
  Sum8 : Sum  Inputs=++--
  Sum9 : Sum  Inputs=+--
  Td1 : Gain  Gain=0.045
  Teeth1 : Gain  Gain=100
  Teeth3 : Gain  Gain=100
  Theta : Outport
  W : Outport  Port=2
  Te : Outport  Port=3
  wires:
  Sum10/1 -> 1/L3/1
  1/L3/1 -> Integrator9/1  "ib_dot"
  Cos1/1 -> Kma5/1, Product9/2
  Tload/1 -> Sum8/4
  Gain2/1 -> Sin5/1
  Sum9/1 -> 1/L2/1
  SignalB/1 -> Sum10/3
  Sum13/1 -> 1/J1/1
  Product8/1 -> 1/Rm2/1, Sum9/2  "ea"
  Product11/1 -> Sum8/2
  Teeth3/1 -> Gain2/1, Cos1/1
  SignalA/1 -> Sum9/1
  Sum11/1 -> Product10/2  "ia-ea/Rm"
  1/Rm3/1 -> Sum12/1
  B1/1 -> Sum13/2
  Integrator7/1 -> Theta/1, Teeth1/1, Teeth3/1  "theta"
  Integrator6/1 -> Kmb1/1, B1/1, Kma3/1, W/1, Integrator7/1  "w"
  Sin4/1 -> Kma4/1, Product8/1
  Integrator8/1 -> Scope6/1, Sum11/1, R2/1  "ia"
  R2/1 -> Sum9/3
  Product9/1 -> 1/Rm3/1, Sum10/2  "eb"
  Kma3/1 -> Product8/2
  Sum12/1 -> Product11/1  "ib-eb/Rm"
  1/Rm2/1 -> Sum11/2
  Kmb1/1 -> Product9/1
  Product10/1 -> Sum8/1  "Tea"
  Integrator9/1 -> Scope6/2, Sum12/2, R3/1  "ib"
  Sum8/1 -> Te/1, Sum13/1  "Te"
  1/J1/1 -> Integrator6/1  "w_dot"
  Kma4/1 -> Product10/1  "-Kmsin(Ntheta)"
  Sin5/1 -> Td1/1
  Kma5/1 -> Product11/2  "Kmcos(Ntheta)"
  1/L2/1 -> Integrator8/1  "ia_dot"
  Teeth1/1 -> Sin4/1
  R3/1 -> Sum10/1
  Td1/1 -> Sum8/3

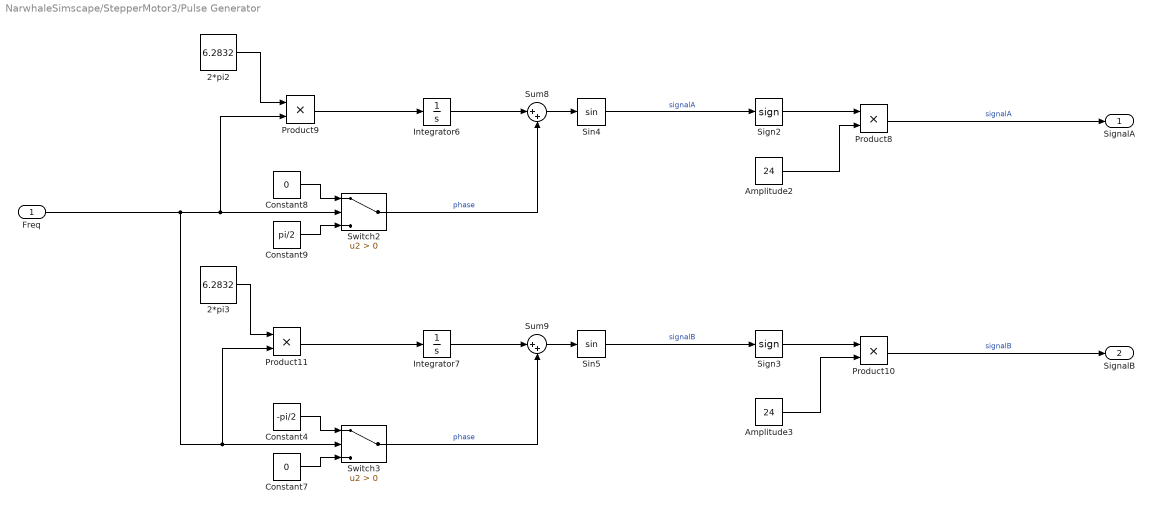
== system NarwhaleSimscape/StepperMotor3/Pulse Generator ==
  Freq : Inport
  2*pi2 : Constant  Value=6.2832
  2*pi3 : Constant  Value=6.2832
  Amplitude2 : Constant  Value=24
  Amplitude3 : Constant  Value=24
  Constant4 : Constant  Value=-pi/2
  Constant7 : Constant  Value=0
  Constant8 : Constant  Value=0
  Constant9 : Constant  Value=pi/2
  Integrator6 : Integrator
  Integrator7 : Integrator
  Product{8..11} (4 alike) : Product
  Sign2 : Signum
  Sign3 : Signum
  Sin4 : Trigonometry
  Sin5 : Trigonometry
  Sum8 : Sum  Inputs=|++
  Sum9 : Sum  Inputs=|++
  Switch2 : Switch  Criteria=u2 > Threshold
  Switch3 : Switch  Criteria=u2 > Threshold
  SignalA : Outport
  SignalB : Outport  Port=2
  wires:
  Product11/1 -> Integrator7/1
  Switch3/1 -> Sum9/2  "phase"
  Sum8/1 -> Sin4/1
  Sign3/1 -> Product10/1
  Integrator7/1 -> Sum9/1
  Freq/1 -> Product11/2, Switch3/2, Product9/2, Switch2/2
  Sin5/1 -> Sign3/1  "signalB"
  Sign2/1 -> Product8/1
  Product10/1 -> SignalB/1  "signalB"
  Product8/1 -> SignalA/1  "signalA"
  Amplitude3/1 -> Product10/2
  Sum9/1 -> Sin5/1
  Amplitude2/1 -> Product8/2
  Integrator6/1 -> Sum8/1
  Constant4/1 -> Switch3/1
  Constant7/1 -> Switch3/3
  2*pi3/1 -> Product11/1
  Switch2/1 -> Sum8/2  "phase"
  Constant9/1 -> Switch2/3
  Constant8/1 -> Switch2/1
  2*pi2/1 -> Product9/1
  Sin4/1 -> Sign2/1  "signalA"
  Product9/1 -> Integrator6/1

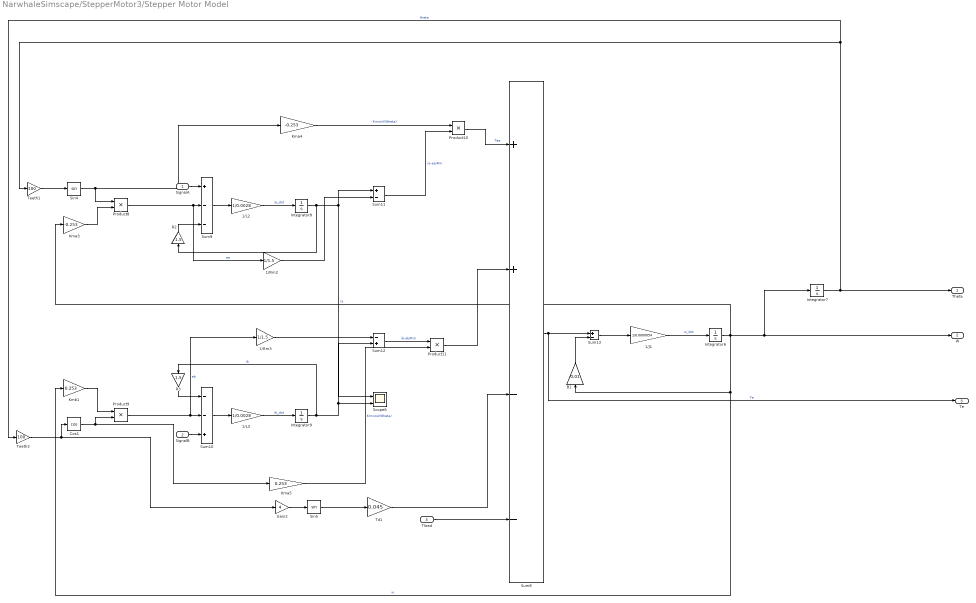
== system NarwhaleSimscape/StepperMotor3/Stepper Motor Model ==
  SignalA : Inport
  SignalB : Inport  Port=2
  Tload : Inport  Port=3
  1/J1 : Gain  Gain=1/0.0000054
  1/L2 : Gain  Gain=1/0.0028
  1/L3 : Gain  Gain=1/0.0028
  1/Rm2 : Gain  Gain=1/1.5
  1/Rm3 : Gain  Gain=1/1.5
  B1 : Gain  Gain=0.01
  Cos1 : Trigonometry  Operator=cos
  Gain2 : Gain  Gain=4
  Integrator{6..9} (4 alike) : Integrator
  Kma3 : Gain  Gain=-0.253
  Kma4 : Gain  Gain=-0.253
  Kma5 : Gain  Gain=0.253
  Kmb1 : Gain  Gain=0.253
  Product{8..11} (4 alike) : Product
  R2 : Gain  Gain=1.5
  R3 : Gain  Gain=1.5
  Scope6 : Scope  NumInputPorts=2
  Sin4 : Trigonometry
  Sin5 : Trigonometry
  Sum10 : Sum  Inputs=--+
  Sum11 : Sum  Inputs=+-
  Sum12 : Sum  Inputs=-+
  Sum13 : Sum  Inputs=+-
  Sum8 : Sum  Inputs=++--
  Sum9 : Sum  Inputs=+--
  Td1 : Gain  Gain=0.045
  Teeth1 : Gain  Gain=100
  Teeth3 : Gain  Gain=100
  Theta : Outport
  W : Outport  Port=2
  Te : Outport  Port=3
  wires:
  Sum10/1 -> 1/L3/1
  1/L3/1 -> Integrator9/1  "ib_dot"
  Cos1/1 -> Kma5/1, Product9/2
  Tload/1 -> Sum8/4
  Gain2/1 -> Sin5/1
  Sum9/1 -> 1/L2/1
  SignalB/1 -> Sum10/3
  Sum13/1 -> 1/J1/1
  Product8/1 -> 1/Rm2/1, Sum9/2  "ea"
  Product11/1 -> Sum8/2
  Teeth3/1 -> Gain2/1, Cos1/1
  SignalA/1 -> Sum9/1
  Sum11/1 -> Product10/2  "ia-ea/Rm"
  1/Rm3/1 -> Sum12/1
  B1/1 -> Sum13/2
  Integrator7/1 -> Theta/1, Teeth1/1, Teeth3/1  "theta"
  Integrator6/1 -> Kmb1/1, B1/1, Kma3/1, W/1, Integrator7/1  "w"
  Sin4/1 -> Kma4/1, Product8/1
  Integrator8/1 -> Scope6/1, Sum11/1, R2/1  "ia"
  R2/1 -> Sum9/3
  Product9/1 -> 1/Rm3/1, Sum10/2  "eb"
  Kma3/1 -> Product8/2
  Sum12/1 -> Product11/1  "ib-eb/Rm"
  1/Rm2/1 -> Sum11/2
  Kmb1/1 -> Product9/1
  Product10/1 -> Sum8/1  "Tea"
  Integrator9/1 -> Scope6/2, Sum12/2, R3/1  "ib"
  Sum8/1 -> Te/1, Sum13/1  "Te"
  1/J1/1 -> Integrator6/1  "w_dot"
  Kma4/1 -> Product10/1  "-Kmsin(Ntheta)"
  Sin5/1 -> Td1/1
  Kma5/1 -> Product11/2  "Kmcos(Ntheta)"
  1/L2/1 -> Integrator8/1  "ia_dot"
  Teeth1/1 -> Sin4/1
  R3/1 -> Sum10/1
  Td1/1 -> Sum8/3

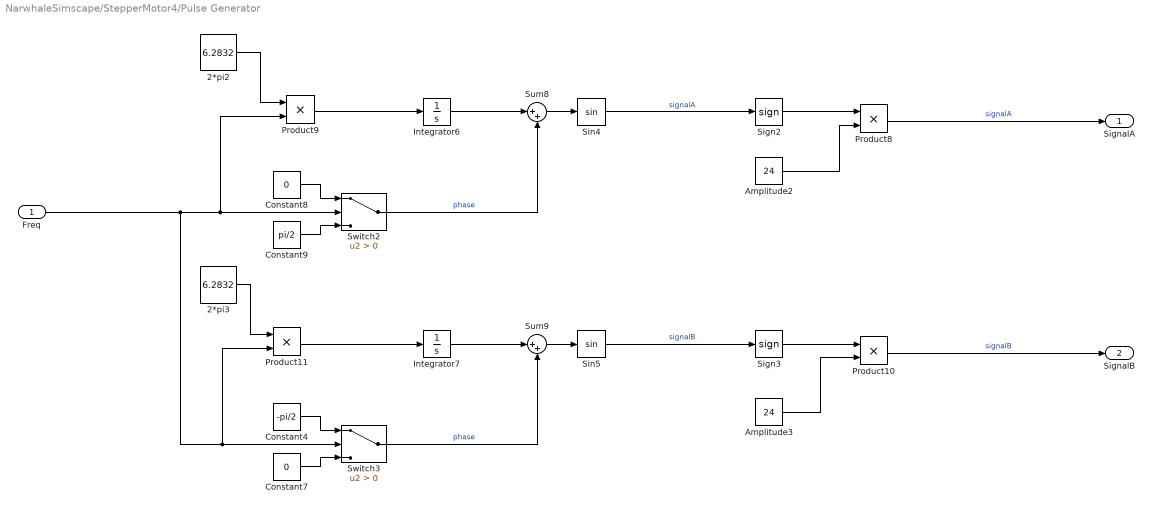
== system NarwhaleSimscape/StepperMotor4/Pulse Generator ==
  Freq : Inport
  2*pi2 : Constant  Value=6.2832
  2*pi3 : Constant  Value=6.2832
  Amplitude2 : Constant  Value=24
  Amplitude3 : Constant  Value=24
  Constant4 : Constant  Value=-pi/2
  Constant7 : Constant  Value=0
  Constant8 : Constant  Value=0
  Constant9 : Constant  Value=pi/2
  Integrator6 : Integrator
  Integrator7 : Integrator
  Product{8..11} (4 alike) : Product
  Sign2 : Signum
  Sign3 : Signum
  Sin4 : Trigonometry
  Sin5 : Trigonometry
  Sum8 : Sum  Inputs=|++
  Sum9 : Sum  Inputs=|++
  Switch2 : Switch  Criteria=u2 > Threshold
  Switch3 : Switch  Criteria=u2 > Threshold
  SignalA : Outport
  SignalB : Outport  Port=2
  wires:
  Product11/1 -> Integrator7/1
  Switch3/1 -> Sum9/2  "phase"
  Sum8/1 -> Sin4/1
  Sign3/1 -> Product10/1
  Integrator7/1 -> Sum9/1
  Freq/1 -> Product11/2, Switch3/2, Product9/2, Switch2/2
  Sin5/1 -> Sign3/1  "signalB"
  Sign2/1 -> Product8/1
  Product10/1 -> SignalB/1  "signalB"
  Product8/1 -> SignalA/1  "signalA"
  Amplitude3/1 -> Product10/2
  Sum9/1 -> Sin5/1
  Amplitude2/1 -> Product8/2
  Integrator6/1 -> Sum8/1
  Constant4/1 -> Switch3/1
  Constant7/1 -> Switch3/3
  2*pi3/1 -> Product11/1
  Switch2/1 -> Sum8/2  "phase"
  Constant9/1 -> Switch2/3
  Constant8/1 -> Switch2/1
  2*pi2/1 -> Product9/1
  Sin4/1 -> Sign2/1  "signalA"
  Product9/1 -> Integrator6/1

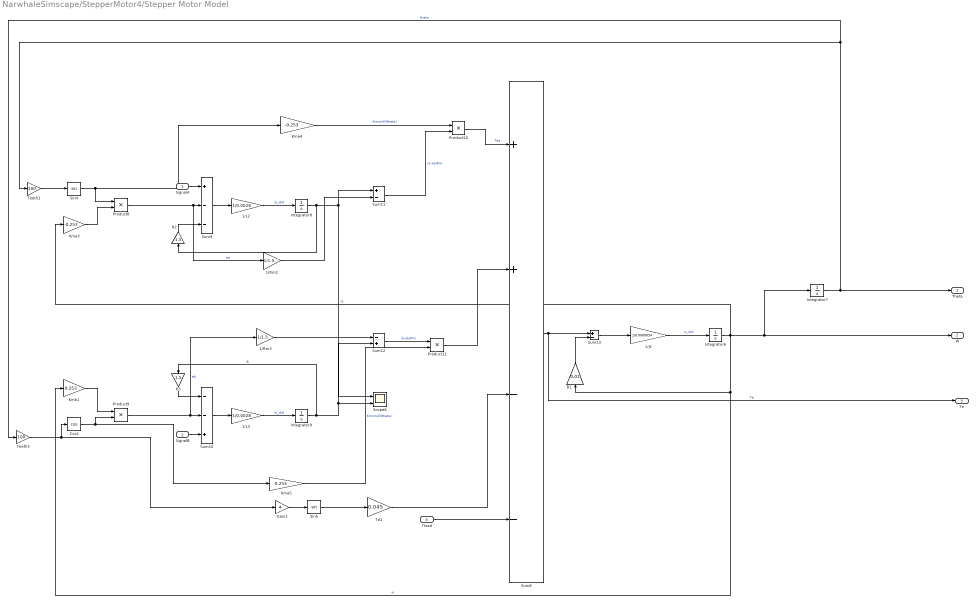
== system NarwhaleSimscape/StepperMotor4/Stepper Motor Model ==
  SignalA : Inport
  SignalB : Inport  Port=2
  Tload : Inport  Port=3
  1/J1 : Gain  Gain=1/0.0000054
  1/L2 : Gain  Gain=1/0.0028
  1/L3 : Gain  Gain=1/0.0028
  1/Rm2 : Gain  Gain=1/1.5
  1/Rm3 : Gain  Gain=1/1.5
  B1 : Gain  Gain=0.01
  Cos1 : Trigonometry  Operator=cos
  Gain2 : Gain  Gain=4
  Integrator{6..9} (4 alike) : Integrator
  Kma3 : Gain  Gain=-0.253
  Kma4 : Gain  Gain=-0.253
  Kma5 : Gain  Gain=0.253
  Kmb1 : Gain  Gain=0.253
  Product{8..11} (4 alike) : Product
  R2 : Gain  Gain=1.5
  R3 : Gain  Gain=1.5
  Scope6 : Scope  NumInputPorts=2
  Sin4 : Trigonometry
  Sin5 : Trigonometry
  Sum10 : Sum  Inputs=--+
  Sum11 : Sum  Inputs=+-
  Sum12 : Sum  Inputs=-+
  Sum13 : Sum  Inputs=+-
  Sum8 : Sum  Inputs=++--
  Sum9 : Sum  Inputs=+--
  Td1 : Gain  Gain=0.045
  Teeth1 : Gain  Gain=100
  Teeth3 : Gain  Gain=100
  Theta : Outport
  W : Outport  Port=2
  Te : Outport  Port=3
  wires:
  Sum10/1 -> 1/L3/1
  1/L3/1 -> Integrator9/1  "ib_dot"
  Cos1/1 -> Kma5/1, Product9/2
  Tload/1 -> Sum8/4
  Gain2/1 -> Sin5/1
  Sum9/1 -> 1/L2/1
  SignalB/1 -> Sum10/3
  Sum13/1 -> 1/J1/1
  Product8/1 -> 1/Rm2/1, Sum9/2  "ea"
  Product11/1 -> Sum8/2
  Teeth3/1 -> Gain2/1, Cos1/1
  SignalA/1 -> Sum9/1
  Sum11/1 -> Product10/2  "ia-ea/Rm"
  1/Rm3/1 -> Sum12/1
  B1/1 -> Sum13/2
  Integrator7/1 -> Theta/1, Teeth1/1, Teeth3/1  "theta"
  Integrator6/1 -> Kmb1/1, B1/1, Kma3/1, W/1, Integrator7/1  "w"
  Sin4/1 -> Kma4/1, Product8/1
  Integrator8/1 -> Scope6/1, Sum11/1, R2/1  "ia"
  R2/1 -> Sum9/3
  Product9/1 -> 1/Rm3/1, Sum10/2  "eb"
  Kma3/1 -> Product8/2
  Sum12/1 -> Product11/1  "ib-eb/Rm"
  1/Rm2/1 -> Sum11/2
  Kmb1/1 -> Product9/1
  Product10/1 -> Sum8/1  "Tea"
  Integrator9/1 -> Scope6/2, Sum12/2, R3/1  "ib"
  Sum8/1 -> Te/1, Sum13/1  "Te"
  1/J1/1 -> Integrator6/1  "w_dot"
  Kma4/1 -> Product10/1  "-Kmsin(Ntheta)"
  Sin5/1 -> Td1/1
  Kma5/1 -> Product11/2  "Kmcos(Ntheta)"
  1/L2/1 -> Integrator8/1  "ia_dot"
  Teeth1/1 -> Sin4/1
  R3/1 -> Sum10/1
  Td1/1 -> Sum8/3
